simulink model "model"  (R2024a)
settings: Solver=FixedStepAuto  StartTime=0.0  StopTime=10e-9  FixedStep=2.5e-12  RelTol=1e-3
libraries: dspsrcs4 x1
settings Model: PauseTimes=1e-9  Creator=fercl  LastModifiedBy=fercl

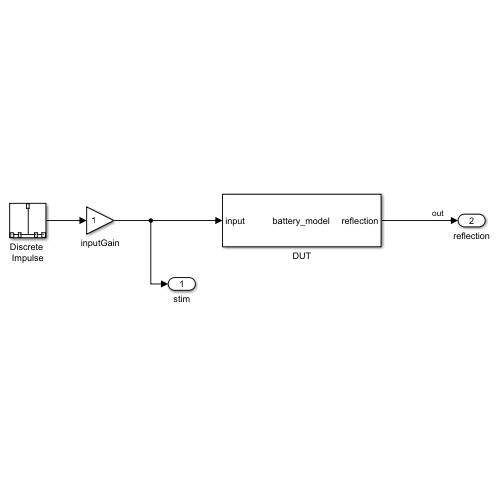
[thumbnail: Simulink's stored preview of the top-level diagram]
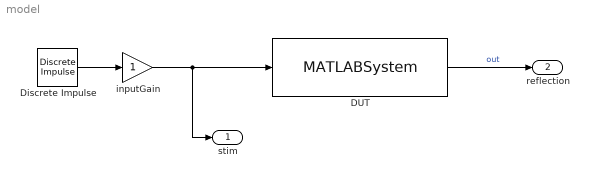
== system model ==
  DUT : MATLABSystem  System=battery_model  NUM_IMPEDANCES=3  REFLECT_COEF=[0.3 0.5 0.7]  PROPAGATION_DELAY=200e-9  STEP_TIME=2.5e-12  DELAY_LENGTH=200  SimulateUsing=Code generation
      mask Type: battery_model
      mask Display:
      | disp('battery_model');
      | port_label('input',1,'input');
      | port_label('output',1,'reflection');
  Discrete Impulse : dspsrcs4/Discrete  Impulse  Delay=0  SampleTime=2.5e-12  FrameSample=1  OutputFrames=off  dataType=double  isSigned=on  wordLen=16  udDataType=sfix(16)  fracBitsMode=Best precision  numFracBits=15  OutDataTypeStr=double  LastOutDataTypeStr=double
  inputGain : Gain
  stim : Outport
  reflection : Outport  Port=2
  wires:
  Discrete Impulse/1 -> inputGain/1
  DUT/1 -> reflection/1  "out"
  inputGain/1 -> stim/1, DUT/1
